simulink model "SolarPVACWithBattery_segmented1"  (R2024a)
settings: Solver=ode23t  StartTime=0.0  StopTime=25  MaxStep=1/(5*solarPlant.converterSwitchingFrequency)  RelTol=1e-3  AbsTol=1e-3
PreLoadFcn:
  | run('SolarPVACWithBatteryData');
undefined symbols (not defined in the file): bms, boost, dcVoltage, maxSoC, maxVdc, minIrrad, minSoC, minVdc, mppttime, olTime, sensor, sigbuilder_block, solarPlant
libraries: simulink x29, nesl_utility x21, fl_lib x19, ee_lib x15, eePwmGenerator x7, SignalEditorBlockLib x2, dspfdesign x1, batteryecm_lib x1, simulink_extras x1
(part 3 of 3)

== system SolarPVACWithBattery_segmented1/MPPT/PO/MPPT/MPPT Algorithm/PerturbationAndObsrvation ==
  note: Both voltage and power is in falling trend
  note: Both voltage and power is in raising trend
  Ipv : Inport
  Vpv : Inport  Port=2
  AND : Logic  IconShape=distinctive  AllPortsSameDT=off  OutDataTypeStr=boolean
  Compare To Constant : simulink/Logic and Bit Operations/Compare To Constant  relop=>=  const=0  OutDataTypeStr=boolean
  Compare To Zero1 : simulink/Logic and Bit Operations/Compare To Zero  relop=>=  OutDataTypeStr=boolean
  Demux : Demux  Outputs=2
  Mux : Mux  Inputs=2
  NOR : Logic  Operator=NOR  IconShape=distinctive  AllPortsSameDT=off  OutDataTypeStr=boolean
  OR : Logic  Operator=OR  IconShape=distinctive  AllPortsSameDT=off  OutDataTypeStr=boolean
  Product : Product
  Product1 : Product
  Subtract : Sum  Inputs=+-
  Subtract4 : Sum  Inputs=-+
  Switch4 : Switch  Criteria=u2 ~= 0  SaturateOnIntegerOverflow=off  InputSameDT=off
  Unit Delay : UnitDelay  InitialCondition=solarPlant.startMPPTValue  SampleTime=1/20000  HasFrameUpgradeWarning=on
  Zero-Order Hold : ZeroOrderHold  SampleTime=solarPlant.timeMPPT
  Vmpp : Outport  VectorParamsAs1DForOutWhenUnconnected=off
  wires:
  NOR/1 -> OR/2
  OR/1 -> Switch4/2
  Compare To Zero1/1 -> AND/2, NOR/2
  AND/1 -> OR/1
  Compare To Constant/1 -> AND/1, NOR/1
  Mux/1 -> Unit Delay/1
  Ipv/1 -> Product1/2, Mux/1
  Demux/1 -> Product/1
  Unit Delay/1 -> Demux/1
  Demux/2 -> Product/2, Subtract4/1  "voltage old"
  Vpv/1 -> Subtract4/2, Product1/1, Mux/2  "voltage now"
  Product1/1 -> Subtract/1  "power now"
  Product/1 -> Subtract/2  "power old"
  Subtract4/1 -> Compare To Zero1/1  "delV"
  Subtract/1 -> Compare To Constant/1  "delPower"
  Switch4/1 -> Zero-Order Hold/1
  [Vdec] -> Switch4/3
  [Vinc] -> Switch4/1
  Zero-Order Hold/1 -> Vmpp/1

== system SolarPVACWithBattery_segmented1/MPPT/Maximum Power Point/MPPT/MPPT Algorithm/IncrementalConductance/If Action Subsystem ==
  In1 : Inport
  Action Port : ActionPort
  Compare To Constant : simulink/Logic and Bit Operations/Compare To Constant  relop===  const=0  OutDataTypeStr=boolean
  Compare To Zero2 : simulink/Logic and Bit Operations/Compare To Zero  relop=>  OutDataTypeStr=boolean
  Set : Outport  VectorParamsAs1DForOutWhenUnconnected=off
  Inc : Outport  Port=2  VectorParamsAs1DForOutWhenUnconnected=off
  wires:
  Compare To Constant/1 -> Set/1  "Yes"
  Compare To Zero2/1 -> Inc/1  "Yes"
  In1/1 -> Compare To Zero2/1, Compare To Constant/1  "delI"

== system SolarPVACWithBattery_segmented1/MPPT/Maximum Power Point/MPPT/MPPT Algorithm/IncrementalConductance/If Action Subsystem1 ==
  delI : Inport
  delV : Inport  Port=2
  Vpv : Inport  Port=3
  Ipv : Inport  Port=4
  Action Port : ActionPort
  Add : Sum
  Compare To Zero : simulink/Logic and Bit Operations/Compare To Zero  relop===  OutDataTypeStr=boolean
  Compare To Zero1 : simulink/Logic and Bit Operations/Compare To Zero  relop=>  OutDataTypeStr=boolean
  Divide : Product  Inputs=*/
  Product : Product
  Set : Outport  VectorParamsAs1DForOutWhenUnconnected=off
  Inc : Outport  Port=2  VectorParamsAs1DForOutWhenUnconnected=off
  wires:
  delI/1 -> Divide/1
  delV/1 -> Divide/2
  Divide/1 -> Product/1
  Add/1 -> Compare To Zero1/1, Compare To Zero/1
  Compare To Zero/1 -> Set/1  "set"
  Vpv/1 -> Product/2
  Product/1 -> Add/1
  Ipv/1 -> Add/2
  Compare To Zero1/1 -> Inc/1  "Increase"

== system SolarPVACWithBattery_segmented1/MPPT/Maximum Power Point1/MPPT/MPPT Algorithm/IncrementalConductance/If Action Subsystem ==
  In1 : Inport
  Action Port : ActionPort
  Compare To Constant : simulink/Logic and Bit Operations/Compare To Constant  relop===  const=0  OutDataTypeStr=boolean
  Compare To Zero2 : simulink/Logic and Bit Operations/Compare To Zero  relop=>  OutDataTypeStr=boolean
  Set : Outport  VectorParamsAs1DForOutWhenUnconnected=off
  Inc : Outport  Port=2  VectorParamsAs1DForOutWhenUnconnected=off
  wires:
  Compare To Constant/1 -> Set/1  "Yes"
  Compare To Zero2/1 -> Inc/1  "Yes"
  In1/1 -> Compare To Zero2/1, Compare To Constant/1  "delI"

== system SolarPVACWithBattery_segmented1/MPPT/Maximum Power Point1/MPPT/MPPT Algorithm/IncrementalConductance/If Action Subsystem1 ==
  delI : Inport
  delV : Inport  Port=2
  Vpv : Inport  Port=3
  Ipv : Inport  Port=4
  Action Port : ActionPort
  Add : Sum
  Compare To Zero : simulink/Logic and Bit Operations/Compare To Zero  relop===  OutDataTypeStr=boolean
  Compare To Zero1 : simulink/Logic and Bit Operations/Compare To Zero  relop=>  OutDataTypeStr=boolean
  Divide : Product  Inputs=*/
  Product : Product
  Set : Outport  VectorParamsAs1DForOutWhenUnconnected=off
  Inc : Outport  Port=2  VectorParamsAs1DForOutWhenUnconnected=off
  wires:
  delI/1 -> Divide/1
  delV/1 -> Divide/2
  Divide/1 -> Product/1
  Add/1 -> Compare To Zero1/1, Compare To Zero/1
  Compare To Zero/1 -> Set/1  "set"
  Vpv/1 -> Product/2
  Product/1 -> Add/1
  Ipv/1 -> Add/2
  Compare To Zero1/1 -> Inc/1  "Increase"

== system SolarPVACWithBattery_segmented1/MPPT/PO/MPPT/MPPT Algorithm/IncrementalConductance/If Action Subsystem ==
  In1 : Inport
  Action Port : ActionPort
  Compare To Constant : simulink/Logic and Bit Operations/Compare To Constant  relop===  const=0  OutDataTypeStr=boolean
  Compare To Zero2 : simulink/Logic and Bit Operations/Compare To Zero  relop=>  OutDataTypeStr=boolean
  Set : Outport  VectorParamsAs1DForOutWhenUnconnected=off
  Inc : Outport  Port=2  VectorParamsAs1DForOutWhenUnconnected=off
  wires:
  Compare To Constant/1 -> Set/1  "Yes"
  Compare To Zero2/1 -> Inc/1  "Yes"
  In1/1 -> Compare To Zero2/1, Compare To Constant/1  "delI"

== system SolarPVACWithBattery_segmented1/MPPT/PO/MPPT/MPPT Algorithm/IncrementalConductance/If Action Subsystem1 ==
  delI : Inport
  delV : Inport  Port=2
  Vpv : Inport  Port=3
  Ipv : Inport  Port=4
  Action Port : ActionPort
  Add : Sum
  Compare To Zero : simulink/Logic and Bit Operations/Compare To Zero  relop===  OutDataTypeStr=boolean
  Compare To Zero1 : simulink/Logic and Bit Operations/Compare To Zero  relop=>  OutDataTypeStr=boolean
  Divide : Product  Inputs=*/
  Product : Product
  Set : Outport  VectorParamsAs1DForOutWhenUnconnected=off
  Inc : Outport  Port=2  VectorParamsAs1DForOutWhenUnconnected=off
  wires:
  delI/1 -> Divide/1
  delV/1 -> Divide/2
  Divide/1 -> Product/1
  Add/1 -> Compare To Zero1/1, Compare To Zero/1
  Compare To Zero/1 -> Set/1  "set"
  Vpv/1 -> Product/2
  Product/1 -> Add/1
  Ipv/1 -> Add/2
  Compare To Zero1/1 -> Inc/1  "Increase"

== matlab function SolarPVACWithBattery_segmented1/MATLAB Function1 ==
  data: i input; q output; x input
function q  = fcn(i,x)

if i >0
    x=x;
    
else
    x=-x;

end

if i> x
    q=0;
else
    q=1;
end

== stateflow chart SolarPVACWithBattery_segmented1/Chart3 ==
  state P10
    entry:
    FC=0;P10=1;
    N=1;Vcon=0;
    exit:
    P10=0;
  state P7
    entry:
    FC=1;P7=1;
    N=1;
    K=300;Vcon=0;
    exit:
    P7=0;
  state P6
    entry:
    FC=1;P6=1;
    N=1;
    K=500;Vcon=0;
    exit:
    P6=0;
  state P8
    entry:
    FC=1;P8=1;
    N=1;
    K=-200;Vcon=0;
    exit:
    P8=0;
  state P9
    entry:
    FC=1;P9=1;
    N=1;
    K=-400;Vcon=0;
    exit:
    P9=0;
  state P4
    entry:
    FC=1;P4=1;
    N=0;
    K=-400;Vcon=0;
    exit:
    P4=0;
  state P3
    entry:
    FC=1;P3=1;
    N=0;
    K=-200;Vcon=0;
    exit:
    P3=0;
  state P2
    entry:
    FC=1;P2=1;
    N=0;K=300;
    Vcon=0;
    exit:
    P2=0;
  state P1
    entry:
    FC=1;P1=1;
    N=0;
    K=500;Vcon=0;
    exit:
    P1=0;
  state P5
    entry:
    FC=0;P5=1;
    N=0;
    Vcon=0;
    exit:
    P5=0;
  state P11
    entry:
    Vcon=1;P11=1;
    FC=0;
    exit:
    P11=0;FC=0;
  P10 -> P6 [order 1] : [soc<7.995 ||PL>1500 ]
  (junction 125) -> P10 : [Irrad<50]
  (junction 133) -> (junction 125)
  P10 -> (junction 127) [order 2]
  (junction 127) -> (junction 126)
  P7 -> P10 [order 4] : [PL<1350]
  P9 -> P10 [order 3] : [PL<1350]
  P8 -> P10 [order 4] : [PL<1350]
  P8 -> P7 [order 1] : [soc<7.9975]
  P7 -> P6 [order 2] : [soc<7.995]
  P8 -> P9 [order 2] : [soc>8.0050]
  P7 -> P8 [order 1] : [soc>8.0025]
  P6 -> P7 [order 1] : [soc>7.9975]
  P9 -> P8 [order 1] : [soc<8.0025]
  P2 -> P7 [order 3] : [Irrad<50]
  P7 -> P2 [order 3] : [Irrad>100]
  P1 -> P6 [order 2] : [Irrad<50]
  P6 -> P1 [order 2] : [Irrad>100]
  P3 -> P8 [order 3] : [Irrad<50]
  P8 -> P3 [order 3] : [Irrad>100]
  P4 -> P9 [order 2] : [Irrad<50]
  P9 -> P4 [order 2] : [Irrad>100]
  P2 -> P1 [order 2] : [soc<7.995]
  P3 -> P4 [order 2] : [soc>8.0050]
  P3 -> P2 [order 1] : [soc<7.9975]
  P1 -> P2 [order 1] : [soc>7.9975]
  P4 -> P3 [order 1] : [soc<8.0025]
  P2 -> P3 [order 1] : [soc>8.0025]
  P4 -> P5 [order 3] : [PL<Ppv+1350]
  P3 -> P5 [order 4] : [PL<Ppv+1350]
  P5 -> P1 [order 1] : [PL>Ppv+1500||soc<7.995||(soc>8.0075&&PL>Ppv)]
  P2 -> P5 [order 4] : [PL<Ppv+1300]
  (junction 126) -> P5 : [Irrad>100]
  P5 -> P11 [order 2] : [soc>8.0075]
  P5 -> (junction 133) [order 3]
  P11 -> P5 : [Vo<97]
  (default) -> P5
  data: soc input; K output; Ppv input; PL input; FC output; N output; Vo input; Vcon output; Irrad input; P1 output; P2 output; P3 output; P4 output; P5 output; P6 output; P7 output; P8 output; P9 output; P10 output; P11 output

== stateflow chart SolarPVACWithBattery_segmented1/Mode Control ==
  state ? [group]
  state aIrrad_minIrrad_ [group]
  note: [Irrad<minIrrad && SoC>minSoC]
  state Mode2_BatCharge_pvMPPT
    entry:
    pvMPPT=1;
    BatCharge=1;
    modeNum=2;
    overload=0;N=0;
    exit:
    pvMPPT=0; BatCharge=0;N=0;
  state Start_Mode
    entry:
    ShutDown = 0;
    loadShutDown = 1;
    pvMPPT=0;
    VoltageControl=1;
    BatIsolate=1;
    modeNum=0;
    overload=0;N=0;
    exit:
    pvMPPT=0;
    BatIsolate=0;N=0;
    VoltageControl=0;
    loadShutDown = 0;
  state Mode5_System_ShutDown
    entry:
    PVoff=1; BatIsolate=1;N=0;
    ShutDown =1; modeNum=5;
    exit:
    ShutDown =0; PVoff=0;
    BatIsolate=0;N=0;
  state Mode1_batIsolated_pvVoltControl
    entry:
    VoltageControl=1; BatIsolate=1;
    modeNum=1;N=0;
    exit:
    VoltageControl=0; BatIsolate=0;N=0;
  state Mode6_pvMPPT_BatCharge_noload
    entry:
    pvMPPT=1; BatCharge=1;
    loadShutDown=1; modeNum=6;
    overload=1;N=0;
    exit:
    loadShutDown=0; pvMPPT=0;
    BatCharge=0;N=0;
  state Mode3_BatDischarge_pvMPPT
    entry:
    pvMPPT=1; BatDischarge=1;
    modeNum=3; overload=0;N=0;
    exit:
    pvMPPT=0;  BatDischarge=0;
    N=0;
  state Mode4_night_mode
    entry:
    PVoff=1; BatDischarge=1;
    modeNum=4;N=1;
    exit:
    PVoff=0; BatDischarge=0;
    N=0;
  Mode2_BatCharge_pvMPPT -> (junction 121) [order 3] : [Irrad<minIrrad &&SoC>7 && LoadPower<0.7]
  Mode2_BatCharge_pvMPPT -> (junction 131) [order 2] : [Vdc < minVdc && SoC>minSoC]
  (junction 121) -> Mode4_night_mode
  (junction 131) -> (junction 154)
  Mode2_BatCharge_pvMPPT -> (junction 117) [order 5] : [Irrad<minIrrad && SoC<minSoC]
  (junction 132) -> Mode2_BatCharge_pvMPPT : [Vdc > 65 && Irrad>minIrrad &&  LoadPower  < 0.9
      | ]
  (junction 117) -> Mode5_System_ShutDown
  (junction 155) -> (junction 132)
  (junction 130) -> Mode2_BatCharge_pvMPPT : [(Irrad >minIrrad && overload==0) || ...
      | (overload==1 && rsflag==1)]
  Mode5_System_ShutDown -> (junction 130)
  Start_Mode -> Mode2_BatCharge_pvMPPT [order 1] : [SoC<minSoC]
  (junction 123) -> Mode2_BatCharge_pvMPPT
  Mode6_pvMPPT_BatCharge_noload -> (junction 123) [order 3] : [rsflag ==1 && Irrad > minIrrad  ...
      | && SoC <= minSoC]
  Mode2_BatCharge_pvMPPT -> (junction 125) [order 4]
  (default) -> Start_Mode
  (junction 125) -> Mode6_pvMPPT_BatCharge_noload : [duration(Vdc<minVdc)>olTime ...
      |  && SoC<minSoC]
  Mode2_BatCharge_pvMPPT -> Mode1_batIsolated_pvVoltControl [order 1] : [(SoC>maxSoC) || ...
      | (duration(Vdc>maxVdc)>olTime)]
  Start_Mode -> Mode3_BatDischarge_pvMPPT [order 2] : [SoC>5]
  Mode1_batIsolated_pvVoltControl -> (junction 126)
  Mode6_pvMPPT_BatCharge_noload -> Mode5_System_ShutDown [order 2] : [(SoC<minSoC && ...
      | Irrad<minIrrad)|| ...
      | SoC>maxSoC]
  (junction 126) -> Mode3_BatDischarge_pvMPPT : [Vdc<minVdc]
  (junction 161) -> Mode5_System_ShutDown
  Mode4_night_mode -> Mode5_System_ShutDown [order 2] : [SoC<minSoC]
  Mode6_pvMPPT_BatCharge_noload -> (junction 127) [order 1] : [SoC>minSoC && rsflag==1]
  (junction 127) -> Mode3_BatDischarge_pvMPPT
  (junction 133) -> Mode6_pvMPPT_BatCharge_noload
  Mode3_BatDischarge_pvMPPT -> (junction 133) [order 2] : [(duration(Vdc<minVdc)>olTime || ...
      |  (SoC<minSoC && Vdc<minVdc)) && Irrad>minIrrad]
  Mode3_BatDischarge_pvMPPT -> (junction 161) [order 3] : [(SoC<minSoC && Irrad<minIrrad) || ( Irrad<minIrrad && duration(Vdc<minVdc)>olTime) ]
  Mode3_BatDischarge_pvMPPT -> (junction 155) [order 1]
  Mode4_night_mode -> Mode3_BatDischarge_pvMPPT [order 1] : [Irrad>minIrrad && LoadPower > 100]
  Mode3_BatDischarge_pvMPPT -> Mode4_night_mode [order 4] : [Irrad<minIrrad && SoC<12]
  (junction 154) -> Mode3_BatDischarge_pvMPPT
  data: Irrad input; Vdc input; SoC input; ShutDown output; maxSoC parameter; maxVdc parameter; minIrrad parameter; minSoC parameter; minVdc parameter; loadShutDown output; VoltageControl output; BatCharge output; BatDischarge output; BatIsolate output; PVoff output; pvMPPT output; modeNum output; rsflag input; overload output; olTime parameter; LoadPower input; N output

== matlab function SolarPVACWithBattery_segmented1/MATLAB Function3 ==
  data: a1 output; a2 output; a3 output; I1 input; I2 input; I3 input; Vcac input; R input; Pa input; Pr2 input; dPa output; Vmpp input; V1 input; V2 input; V3 input; q output; q input; N input
function [a1,a2,a3,dPa,q]   = fcn(I1,I2,I3,Vcac,R,Pa,Pr2, Vmpp, V1,V2,V3,q,N)

VdC=100;
L1=0.0797;%0.0021;
L2=0.2677;%0.0021;
L3=0.1063;%6.8962e-4;
C=0.015;
%V2=0;
%I2=0;

% Lmd2=100;
% Lmd30=10000;
% Lmd31=500;
% Lmd4=500;
Lmd4=500;

dPa=-Lmd4*(Vcac-VdC);

if N == 0
Id1=V1*I1/Vmpp;
Id2=Pr2/V2;
Id3=(Pa-V1*Id1-V2*Id2)/V3;

hn=0.5*(L1*I1*I1+L2*I2*I2+L3*I3+C*Vcac*Vcac);
dhn=V1*I1+V2*I2+V3*I3-Vcac*Vcac/R;

hdn= 0.5*(L1*Id1*Id1+L2*Id2*Id2+L3*Id3*Id3)+0.5*C*VdC*VdC;
dhdn= 0;%V1*Id1+V2*Id2+V3*Id3-VdC*VdC/R;
ddhdn = 0;

dId1=0;
dId2=0;
dId3=0;



if q == 1 %BOOOSST
    Lmd1=100;
Lmd2=100;
Lmd30=4000;
Lmd31=500;
a1=(L1/Vcac)*((Vcac-V1)/L1-Lmd1*(I1-Id1)+dId1);
a2=(L2/Vcac)*((Vcac-V2)/L2-Lmd2*(I2-Id2)+dId2);
    a3=inv(V3*Vcac/L3+2*Vcac*I3/(R*C))*...
        (-(V1*(V1-Vcac)/L1+V2*(V2-Vcac)/L2+V3*(V3-Vcac)/L3)+...
        2*(Vcac/R)*((I1+I2+I3)/C-Vcac/(R*C))-...
        (V1*Vcac/L1+2*Vcac*I1/(R*C))*a1-(V2*Vcac/L2+2*Vcac*I2/(R*C))*a2...
        -Lmd30*(hn-hdn)-Lmd31*(dhn-dhdn)+ddhdn...
        );

else
    Lmd1=1000;
Lmd2=1000;
Lmd30=20000;
Lmd31=500;
    a1=(L1/Vcac)*((Vcac-V1)/L1-Lmd1*(I1-Id1)+dId1);
a2=(L2/Vcac)*((Vcac-V2)/L2-Lmd2*(I2-Id2)+dId2);
    a3=inv(V3*Vcac/L3+2*Vcac*I3/(R*C))*...
        ((V1*(V1-Vcac)/L1+V3*(V3)/L3+V2*(V2-Vcac)/L2)-...
        2*(Vcac/R)*((I1+I2)/C-Vcac/(R*C))+...
        (V1*Vcac/L1+2*Vcac*I1/(R*C))*a1+(V2*Vcac/L2+2*Vcac*I2/(R*C))*a2...
        +Lmd30*(hn-hdn)+Lmd31*(dhn-dhdn)-ddhdn...
        );
end

else
Id1=0;
Id2=Pr2/V2;
Id3=(Pa-V1*Id1-V2*Id2)/V3;

hn=0.5*(0+L2*I2*I2+L3*I3+C*Vcac*Vcac);
dhn=0+V2*I2+V3*I3-Vcac*Vcac/R;

hdn= 0.5*(0+L2*Id2*Id2+L3*Id3*Id3)+0.5*C*VdC*VdC;
dhdn= 0;%V1*Id1+V2*Id2+V3*Id3-VdC*VdC/R;
ddhdn = 0;

dId1=0;
dId2=0;
dId3=0;



if q == 1 %BOOOSST
    Lmd1=100;
Lmd2=500;
Lmd30=10000;
Lmd31=500;
a1=0;
a2=(L2/Vcac)*((Vcac-V2)/L2-Lmd2*(I2-Id2)+dId2);
    a3=inv(V3*Vcac/L3+2*Vcac*I3/(R*C))*...
        (-(0+V2*(V2-Vcac)/L2+V3*(V3-Vcac)/L3)+...
        2*(Vcac/R)*((0+I2+I3)/C-Vcac/(R*C))-...
        (0)*a1-(V2*Vcac/L2+2*Vcac*I2/(R*C))*a2...
        -Lmd30*(hn-hdn)-Lmd31*(dhn-dhdn)+ddhdn...
        );



else
    Lmd1=100;
Lmd2=500;
Lmd30=10000;
Lmd31=500;
    a1=0;
a2=(L2/Vcac)*((Vcac-V2)/L2-Lmd2*(I2-Id2)+dId2);
    a3=inv(V3*Vcac/L3+2*Vcac*I3/(R*C))*...
        ((0+V3*(V3)/L3+V2*(V2-Vcac)/L2)-...
        2*(Vcac/R)*((0+I2)/C-Vcac/(R*C))+...
        (0)*a1+(V2*Vcac/L2+2*Vcac*I2/(R*C))*a2...
        +Lmd30*(hn-hdn)+Lmd31*(dhn-dhdn)-ddhdn...
        );
end
end

== matlab function SolarPVACWithBattery_segmented1/PV+FC+Batt/PV_FC_Bat ==
  data: Lmd1 input; Lmd2 input; Lmd30 input; Lmd31 input; a1 output; a2 output; a3 output; I1 input; I2 input; I3 input; Id2 input; dId2 input; Id3 input; dId3 input; Vcac input; R input; Vmpp input; V1 input; V2 input; V3 input; q input; FCs input; PVs input
function [a1,a2,a3]   = fcn(Lmd1,Lmd2,Lmd30,Lmd31,I1,I2,I3,Id2,dId2,Id3,dId3,Vcac,R, Vmpp, V1,V2,V3,q,FCs,PVs)

VdC=100;
L1=0.0797;
L2=0.2677;
L3=2e-3;%6.8962e-3;
C=0.015;
%V2=0;
%I2=0;

% Lmd2=100;
% Lmd30=10000;
% Lmd31=500;
% Lmd4=500;



if PVs==0
Id1=0;
else
Id1=V1*I1/1/Vmpp;
end

if FCs==0
Id2=0;
dId2=0;
else
Id2=Id2;
end
Id3=Id3;

hn=0.5*(L1*I1*I1+L2*I2*I2+L3*I3+C*Vcac*Vcac);
dhn=V1*I1+V2*I2+V3*I3-Vcac*Vcac/R;

hdn= 0.5*(L1*Id1*Id1+L2*Id2*Id2+L3*Id3*Id3)+0.5*C*VdC*VdC;
dhdn= V1*Id1+V2*Id2+V3*Id3-VdC*VdC/R;
ddhdn = V2*dId2+V3*dId3;

dId1=0;
%dId2=0;
%dId3=0;

    Lmd1=Lmd1;
Lmd2=Lmd2;
Lmd30=Lmd30;
Lmd31=Lmd31;
   


if q == 1 %BOOOSST

if PVs==0

a1=0;
else

a1=(L1/Vcac)*((Vcac-V1)/L1-Lmd1*(I1-Id1)+dId1);
end

if FCs==0
a2=0;
else
a2=(L2/Vcac)*((Vcac-V2)/L2-Lmd2*(I2-Id2)+dId2);
end
    a3=inv(V3*Vcac/L3+2*Vcac*I3/(R*C))*...
        (-(V1*(V1-Vcac)/L1+V2*(V2-Vcac)/L2+V3*(V3-Vcac)/L3)+...
        2*(Vcac/R)*((I1+I2+I3)/C-Vcac/(R*C))-...
        (V1*Vcac/L1+2*Vcac*I1/(R*C))*a1/1-(V2*Vcac/L2+2*Vcac*I2/(R*C))*a2/1 ...
       -Lmd30*(hn-hdn)-Lmd31*(dhn-dhdn)+ddhdn...
        );



else

if PVs==0
a1=0;
else
a1=(L1/Vcac)*((Vcac-V1)/L1-Lmd1*(I1-Id1)+dId1);
end

if FCs==0
a2=0;
else
a2=(L2/Vcac)*((Vcac-V2)/L2-Lmd2*(I2-Id2)+dId2);
end
    a3=inv(V3*Vcac/L3+2*Vcac*I3/(R*C))*...
        ((V1*(V1-Vcac)/L1+V3*(V3)/L3+V2*(V2-Vcac)/L2)-...
        2*(Vcac/R)*((I1+I2)/C-Vcac/(R*C))+...
        (V1*Vcac/L1+2*Vcac*I1/(R*C))*a1/1+(V2*Vcac/L2+2*Vcac*I2/(R*C))*a2/1 ...
        +Lmd30*(hn-hdn)+Lmd31*(dhn-dhdn)-ddhdn...
        );
end

== matlab function SolarPVACWithBattery_segmented1/Battery Discharging1/MATLAB Function ==
  data: dE input; u output; PL input; PFCo input; PPVo input; Pbatlim input
function u = fcn(dE, PL,PFCo, PPVo,Pbatlim)

%u = 2*Pbatlim*(1-sqrt((1-(dE+PL-PFCo-PPVo)/Pbatlim)));

if (1-(dE+PL-PFCo-PPVo)/Pbatlim) < 0
    u = 0;
else
   u = 2*Pbatlim*(1-sqrt((1-(dE+PL-PFCo-PPVo)/Pbatlim)));
end

== matlab function SolarPVACWithBattery_segmented1/PV+FC+Batt/MATLAB Function4 ==
  data: q input; a1 output; a input; a2 output
function [a1,a2] = fcn(q,a)

if q == 1
    a1=a;
    a2=0;
else
    a1=0;
    a2=a;

end

== matlab function SolarPVACWithBattery_segmented1/PV+FC+Batt/Constant Voltage/PV_FC_Bat ==
  data: Lmd30 input; Lmd31 input; a1 output; I1 input; Id3 input; dId3 input; Vcac input; R input; V1 input
function a1    = fcn(Lmd30,Lmd31,I1,Id3,dId3,Vcac,R, V1)

VdC=100;
L1=0.0797;
C=0.015;
%V2=0;
%I2=0;

% Lmd2=100;
% Lmd30=10000;
% Lmd31=500;
% Lmd4=500;

Id1=Id3;
dId1=dId3;

hn=0.5*(L1*I1*I1+C*Vcac*Vcac);
dhn=V1*I1-Vcac*Vcac/R;

hdn= 0.5*(L1*Id1*Id1)+0.5*C*VdC*VdC;
dhdn= V1*Id1-VdC*VdC/R;
ddhdn = V1*dId1;


a1=inv(V1*Vcac/L1+2*Vcac*I1/(R*C))*...
        (-(V1*(V1-Vcac)/L1+...
        2*(Vcac/R)*((I1)/C-Vcac/(R*C))...
       -Lmd30*(hn-hdn)-Lmd31*(dhn-dhdn)+ddhdn));
